simulink library "mech_stewart_control_deriv"  (Simulink 6.0)
settings: Solver=ode45  SolverMode=SingleTasking  StartTime=0.0  StopTime=10.0  RelTol=1e-3
undefined symbols (not defined in the file or in its folder): transfer_denom, transfer_num
libraries: mech_stewart_control_deriv x1
settings Model: Creator=batserve  LastModifiedBy=batserve  ExtModeAutoUpdateStatusClock=off
settings OptimizationCC: BooleanDataType=off
settings DebuggingCC: SolverPrmCheckMsg=none
settings HardwareCC: TargetUnknown=on

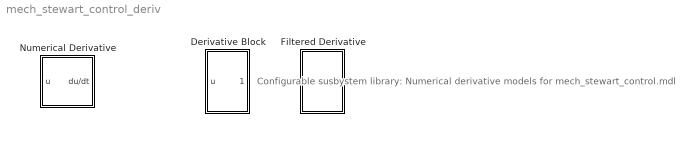
== system mech_stewart_control_deriv ==
  note: Configurable susbystem library:
      | Numerical derivative models for
      | mech_stewart_control.mdl
  Derivative Block : Subsystem
  Filtered Derivative : Subsystem
  "Numerical Derivative " : Subsystem  BlockChoice=Derivative Block
      settings: TemplateBlock=self  MemberBlocks=Derivative Block,Filtered Derivative

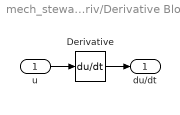
== system mech_stewart_control_deriv/Derivative Block ==
  u : Inport  Port=1  LatchInput=off
  Derivative : Derivative
  du/dt : Outport
  wires:
  Derivative/1 -> du/dt/1
  u/1 -> Derivative/1

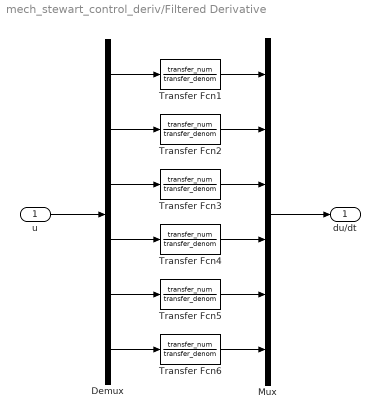
== system mech_stewart_control_deriv/Filtered Derivative ==
  u : Inport  Port=1  LatchInput=off
  Demux : Demux  Outputs=6
  Mux : Mux  Inputs=6
  Transfer Fcn{1..6} (6 alike) : TransferFcn  Numerator=transfer_num  Denominator=transfer_denom
  du/dt : Outport
  wires:
  Mux/1 -> du/dt/1
  u/1 -> Demux/1
  Demux/1 -> Transfer Fcn1/1
  Transfer Fcn1/1 -> Mux/1
  Demux/2 -> Transfer Fcn2/1
  Transfer Fcn2/1 -> Mux/2
  Demux/3 -> Transfer Fcn3/1
  Transfer Fcn3/1 -> Mux/3
  Demux/4 -> Transfer Fcn4/1
  Transfer Fcn4/1 -> Mux/4
  Demux/5 -> Transfer Fcn5/1
  Transfer Fcn5/1 -> Mux/5
  Demux/6 -> Transfer Fcn6/1
  Transfer Fcn6/1 -> Mux/6

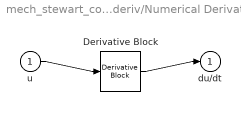
== system mech_stewart_control_deriv/Numerical Derivative  ==
  u : Inport  Port=1  LatchInput=off
  Derivative Block : mech_stewart_control_deriv/Derivative Block
  du/dt : Outport
  wires:
  u/1 -> Derivative Block/1
  Derivative Block/1 -> du/dt/1
